simulink model "MEX_MDL_UDP_test"  (R2022b)
settings: Solver=VariableStepAuto  StartTime=0.0  StopTime=10.0  RelTol=1e-3
libraries: gmp_sil_core x1
settings Model: Creator=javnson  LastModifiedBy=javnson

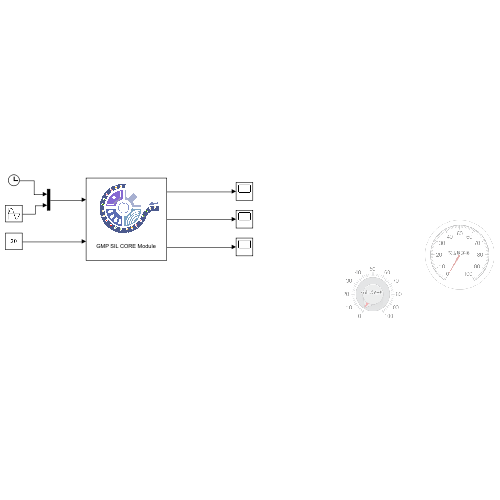
[thumbnail: Simulink's stored preview of the top-level diagram]
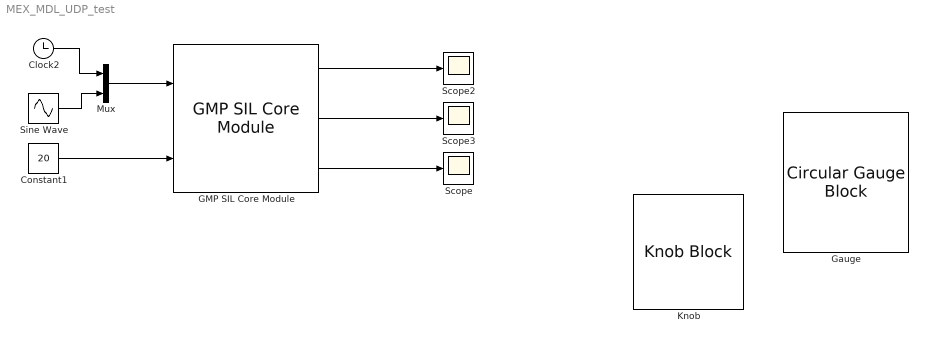
== system MEX_MDL_UDP_test ==
  Clock2 : Clock
  Constant1 : Constant  Value=20
  GMP SIL Core Module : gmp_sil_core/GMP SIL Core Module  MaskPackedDataTypes={'double','double'}  MaskPackedDataSizes={[2],[1]}  MaskUnpackedDataTypes={'double','double','double'}  MaskUnpackedDataSizes={[1],[1],[1]}  MaskAlignment=1  MaskHostAddr='127.0.0.1'  MaskMsgTxPort=12300  MaskMsgRxPort=12301  MaskCmdTxPort=12302  MaskCmdRxPort=12303
      settings: SourceProductName=GMP Utilities Library
  Gauge : CircularGaugeBlock
  Knob : KnobBlock
  Mux : Mux  Inputs=2
  Scope : Scope
  Scope2 : Scope
  Scope3 : Scope
  Sine Wave : Sin  SampleTime=0
  wires:
  GMP SIL Core Module/2 -> Scope3/1
  GMP SIL Core Module/1 -> Scope2/1
  Constant1/1 -> GMP SIL Core Module/2
  GMP SIL Core Module/3 -> Scope/1
  Clock2/1 -> Mux/1
  Mux/1 -> GMP SIL Core Module/1
  Sine Wave/1 -> Mux/2
